simulink model "SimscapePlantModels"  (R2026b)
settings: Solver=VariableStepAuto
undefined symbols (not defined in the file): PlntTrnsfrCaseAxlSpdLock, PlntTrnsfrCaseTrqSplitRatio
libraries: simulink x2, nesl_utility x2
settings Model: ModifiedByFormat=The MathWorks, Inc.  Creator=The MathWorks, Inc.  LastModifiedBy=The MathWorks, Inc.

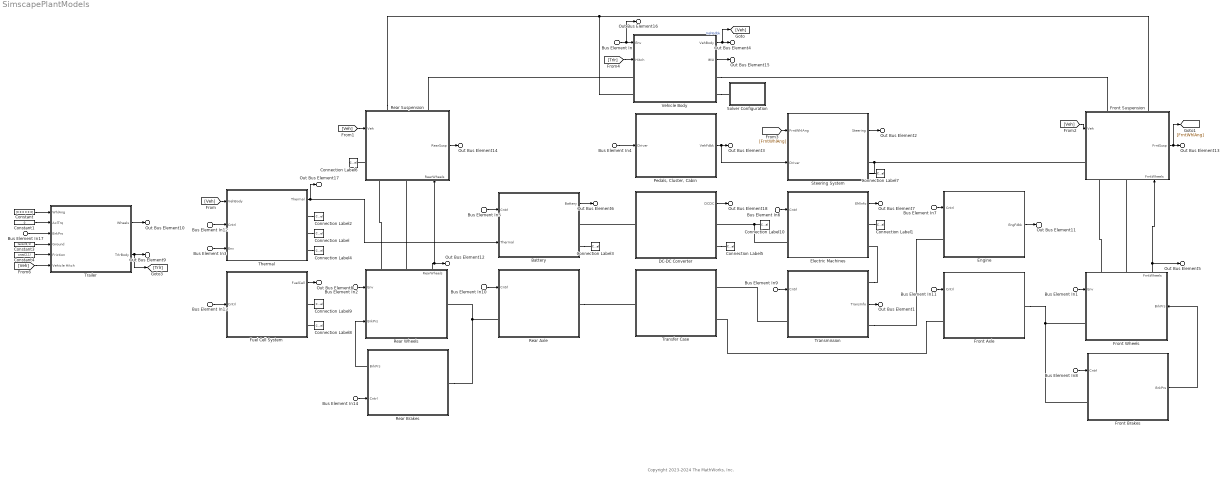
== system SimscapePlantModels ==
  note: Copyright 2023-2024 The MathWorks, Inc.
  Bus Element In{,1..3} (4 alike) : Inport  PortName=Env
  Bus Element In4 : Inport  Port=2  PortName=Driver
  Bus Element In{5..14} (10 alike) : Inport  Port=3  PortName=Cntrl
  Bus Element In17 : Inport  Port=3  PortName=Cntrl  Element=Vcu.VcuTrlrBrkPrsCmd
  Battery : Subsystem  Variant=on  VariantChoicesSpecifier={'BatteryMappedSSC', 'DetailedBatteryModel', 'NoBattery'}  VariantControlMode=label  VariantControl=Battery  LabelModeActiveChoice=NoBattery
      mask Display: image('Battery.png'); % Use "Edit Image" on toolstrip to change.
  Connection Label : ConnectionLabel  Label=ThrmEM
  Connection Label1 : ConnectionLabel  Label=ThrmEM
  Connection Label10 : ConnectionLabel  Label=HVDC
  Connection Label2 : ConnectionLabel  Label=ThrmBatt
  Connection Label3 : ConnectionLabel  Label=ThrmBatt
  Connection Label4 : ConnectionLabel  Label=ThrmPwrE
  Connection Label5 : ConnectionLabel  Label=ThrmPwrE
  Connection Label6 : ConnectionLabel  Label=Steer
  Connection Label7 : ConnectionLabel  Label=Steer
  Connection Label8 : ConnectionLabel  Label=ThrmPwrE
  Connection Label9 : ConnectionLabel  Label=HVDC
  Constant : Constant  Value=[0 0 0 0 0 0]
  Constant1 : Constant  Value=0
  Constant3 : Constant  Value=zeros(2,1)
  Constant4 : Constant  Value=ones(2,1)
  DC-DC Converter : Subsystem  Variant=on  VariantChoicesSpecifier={'DCDCConverterSSC', 'HVDCPassThroughSSC', 'NoDCDCConverter'}  VariantControlMode=label  VariantControl=DC-DC Converter  LabelModeActiveChoice=NoDCDCConverter
      mask Display: image('DCDCConverter.png'); % Use "Edit Image" on toolstrip to change.
  Electric Machines : Subsystem  Variant=on  VariantChoicesSpecifier={'s1EMSSC', 's2EMSSC', 's3EMSSC', 's4EMSSC', 'NoEM'}  VariantControlMode=label  VariantControl=Electric Machines  LabelModeActiveChoice=NoEM
      mask Display: image('Motor.png'); % Use "Edit Image" on toolstrip to change.
  Engine : Subsystem  Variant=on  VariantChoicesSpecifier={'FMUEngineSSC', 'NoEngine', 'SimpleEngineSSC'}  VariantControlMode=label  VariantControl=Engine  LabelModeActiveChoice=SimpleEngineSSC
      settings: PortSchema="{\"entries\":[{\"content\":{\"sides\":[{\"content\":{\"connectorIds\":[\"Out1\"]},\"type\":\"ConnectorPlacement.EquallySpacedRectSide\",\"uuid\":\"a3b8b5c3-27e7-4b20-ab88-ee45fcc797bf\"},{\"content\":{\"connectorIds\":[\"In1\",\"RConn1\"],\"side\":\"RIGHT\"},\"type\":\"ConnectorPlacement.EquallySpacedRectSide\",\"uuid\":\"6bc1f60e-7c62-435c-b993-228d775a2fb7\"},{\"content\":{\"side\":\"TOP\"},\"type\":\"ConnectorPlacement.EquallySpacedRectSide\",\"uuid\":\"10043785-7be0-4314-a245-133c898806ac\"}]},\"type\":\"ConnectorPlacement.EquallySpacedConnector\",\"uuid\":\"16b8f5d8-ca71-4d51-812a-2d43fab8268d\"}],\"packageUris\":[\"http://schema.mathworks.com/mf0/Connector/R2020b\"],\"version\":\"1.0\"}"
      mask Display: image('Engine.png'); % Use "Edit Image" on toolstrip to change.
  Front Axle : Subsystem  Variant=on  VariantChoicesSpecifier={'DualEMDriveFrontSSC', 'LimitedSlipDifferentialSSC', 'NoDifferentialFrontSSC', 'OpenDifferentialSSC'}  VariantControlMode=label  VariantControl=Front Axle  LabelModeActiveChoice=OpenDifferentialSSC
      mask Display: image('Differential.png'); % Use "Edit Image" on toolstrip to change.
  Front Brakes : Subsystem  Variant=on  VariantControlMode=label  LabelModeActiveChoice=BrakingHydraulicsDiscBrakesFrontSSC
      mask Display: image('Caliper.png');
  Front Suspension : Subsystem  Variant=on  VariantChoicesSpecifier={'NoSuspensionFrontSSC', 'MultibodySuspensionFrontSSC'}  VariantControlMode=label  VariantControl=Front Suspension  LabelModeActiveChoice=NoSuspensionFrontSSC
      settings: PortSchema="{\"entries\":[{\"content\":{\"sides\":[{\"content\":{\"connectorIds\":[\"In1\",\"LConn1\"]},\"type\":\"ConnectorPlacement.EquallySpacedRectSide\",\"uuid\":\"36495ae3-e41e-45b1-8235-92554da8a481\"},{\"content\":{\"connectorIds\":[\"Out1\"],\"side\":\"RIGHT\"},\"type\":\"ConnectorPlacement.EquallySpacedRectSide\",\"uuid\":\"e9a47a73-fb93-4125-a24a-a3cc868721b9\"},{\"content\":{\"connectorIds\":[\"LConn2\",\"LConn3\"],\"side\":\"TOP\"},\"type\":\"ConnectorPlacement.EquallySpacedRectSide\",\"uuid\":\"5a383699-364e-4237-a1a1-da409ccbe0dd\"},{\"content\":{\"connectorIds\":[\"RConn1\",\"RConn2\",\"In2\"],\"side\":\"BOTTOM\"},\"type\":\"ConnectorPlacement.EquallySpacedRectSide\",\"uuid\":\"52f047b1-27f7-43e7-8630-25f9b0ada97f\"}]},\"type\":\"ConnectorPlacement.EquallySpacedConnector\",\"uuid\":\"71c041fb-1ceb-419f-94dc-cf2d7d471e97\"}],\"packageUris\":[\"http://schema.mathworks.com/mf0/Connector/R2020b\"],\"version\":\"1.0\"}"
      mask Display: image('SimpleSusp.png'); % Use "Edit Image" on toolstrip to change.
  Front Wheels : Subsystem  Variant=on  VariantChoicesSpecifier={'MFTiresLongitudinalFrontSSC', 'MFTiresMultibodyFrontSSC'}  VariantControlMode=label  VariantControl=Front Wheels  LabelModeActiveChoice=MFTiresLongitudinalFrontSSC
      settings: PortSchema="{\"entries\":[{\"content\":{\"sides\":[{\"content\":{\"connectorIds\":[\"In1\",\"LConn1\"]},\"type\":\"ConnectorPlacement.EquallySpacedRectSide\",\"uuid\":\"18116c41-4c85-4964-ba51-5bd2d68de1c0\"},{\"content\":{\"connectorIds\":[\"In2\"],\"side\":\"RIGHT\"},\"type\":\"ConnectorPlacement.EquallySpacedRectSide\",\"uuid\":\"ed8f79d6-b842-45c2-9629-e45b4856155a\"},{\"content\":{\"connectorIds\":[\"LConn2\",\"LConn3\",\"Out1\"],\"side\":\"TOP\"},\"type\":\"ConnectorPlacement.EquallySpacedRectSide\",\"uuid\":\"6d0f4b93-eb24-4fe5-bb44-e27d25281d66\"}]},\"type\":\"ConnectorPlacement.EquallySpacedConnector\",\"uuid\":\"784a74eb-5e74-45d7-9868-3d9308da2017\"}],\"packageUris\":[\"http://schema.mathworks.com/mf0/Connector/R2020b\"],\"version\":\"1.0\"}"
      mask Display: image('TirewithNoneBrake.png'); % Use "Edit Image" on toolstrip to change.
  Fuel Cell System : Subsystem  Variant=on  VariantControlMode=label  LabelModeActiveChoice=NoFuelCell
  "Pedals, Cluster, Cabin" : Subsystem
  Rear Axle : Subsystem  Variant=on  VariantChoicesSpecifier={'DualEMDriveRear3EMSSC', 'DualEMDriveRear4EMSSC', 'LimitedSlipDifferential2SSC', 'NoDifferentialRearSSC', 'OpenDifferential2SSC'}  VariantControlMode=label  VariantControl=Rear Axle  LabelModeActiveChoice=NoDifferentialRearSSC
      settings: PortSchema="{\"entries\":[{\"content\":{\"sides\":[{\"content\":{\"connectorIds\":[\"LConn1\"]},\"type\":\"ConnectorPlacement.EquallySpacedRectSide\",\"uuid\":\"65d99f67-05a2-47e2-8294-9f529f1023b0\"},{\"content\":{\"connectorIds\":[\"In1\",\"RConn1\"],\"side\":\"RIGHT\"},\"type\":\"ConnectorPlacement.EquallySpacedRectSide\",\"uuid\":\"aa6e28a2-60ee-49c7-b0d1-af08bbc364e9\"},{\"content\":{\"side\":\"TOP\"},\"type\":\"ConnectorPlacement.EquallySpacedRectSide\",\"uuid\":\"5c87d57e-c88d-4b62-ab09-b2529f55e131\"}]},\"type\":\"ConnectorPlacement.EquallySpacedConnector\",\"uuid\":\"05d2764b-b8a6-49cf-a5f1-fcd990b4e9b6\"}],\"packageUris\":[\"http://schema.mathworks.com/mf0/Connector/R2020b\"],\"version\":\"1.0\"}"
      mask Display: image('Differential.png'); % Use "Edit Image" on toolstrip to change.
  Rear Brakes : Subsystem  Variant=on  VariantControlMode=label  LabelModeActiveChoice=BrakingHydraulicsDiscBrakesRearSSC
      settings: PortSchema="{\"entries\":[{\"content\":{\"sides\":[{\"content\":{\"connectorIds\":[\"Out1\",\"In1\"]},\"type\":\"ConnectorPlacement.EquallySpacedRectSide\",\"uuid\":\"1a344f8a-3021-4136-9b8c-8b822c978ed0\"},{\"content\":{\"connectorIds\":[\"RConn1\"],\"side\":\"RIGHT\"},\"type\":\"ConnectorPlacement.EquallySpacedRectSide\",\"uuid\":\"18adbbc3-2fb5-4373-b77a-b21e81530fc9\"},{\"content\":{\"side\":\"TOP\"},\"type\":\"ConnectorPlacement.EquallySpacedRectSide\",\"uuid\":\"fb378fea-1867-4c5a-9e78-cb47ca632c79\"}]},\"type\":\"ConnectorPlacement.EquallySpacedConnector\",\"uuid\":\"a08d4fdb-0a7f-495f-99ba-67ccd9fceaa4\"}],\"packageUris\":[\"http://schema.mathworks.com/mf0/Connector/R2020b\"],\"version\":\"1.0\"}"
      mask Display: image('Caliper.png');
  Rear Suspension : Subsystem  Variant=on  VariantChoicesSpecifier={'NoSuspensionRearSSC', 'MultibodySuspensionRearSSC'}  VariantControlMode=label  VariantControl=Rear Suspension  LabelModeActiveChoice=NoSuspensionRearSSC
      settings: PortSchema="{\"entries\":[{\"content\":{\"sides\":[{\"content\":{\"connectorIds\":[\"In1\",\"LConn1\"]},\"type\":\"ConnectorPlacement.EquallySpacedRectSide\",\"uuid\":\"36495ae3-e41e-45b1-8235-92554da8a481\"},{\"content\":{\"connectorIds\":[\"Out1\"],\"side\":\"RIGHT\"},\"type\":\"ConnectorPlacement.EquallySpacedRectSide\",\"uuid\":\"e9a47a73-fb93-4125-a24a-a3cc868721b9\"},{\"content\":{\"connectorIds\":[\"LConn2\",\"LConn3\"],\"side\":\"TOP\"},\"type\":\"ConnectorPlacement.EquallySpacedRectSide\",\"uuid\":\"5a383699-364e-4237-a1a1-da409ccbe0dd\"},{\"content\":{\"connectorIds\":[\"RConn1\",\"RConn2\",\"In2\"],\"side\":\"BOTTOM\"},\"type\":\"ConnectorPlacement.EquallySpacedRectSide\",\"uuid\":\"f9ad9365-a105-4ce1-87dd-14cbc5e9d7d0\"}]},\"type\":\"ConnectorPlacement.EquallySpacedConnector\",\"uuid\":\"71c041fb-1ceb-419f-94dc-cf2d7d471e97\"}],\"packageUris\":[\"http://schema.mathworks.com/mf0/Connector/R2020b\"],\"version\":\"1.0\"}"
      mask Display: image('SimpleSusp.png'); % Use "Edit Image" on toolstrip to change.
  Rear Wheels : Subsystem  Variant=on  VariantChoicesSpecifier={'MFTiresLongitudinalRearSSC', 'MFTiresMultibodyRearSSC'}  VariantControlMode=label  VariantControl=Rear Wheels  LabelModeActiveChoice=MFTiresLongitudinalRearSSC
      settings: PortSchema="{\"entries\":[{\"content\":{\"sides\":[{\"content\":{\"connectorIds\":[\"LConn1\"]},\"type\":\"ConnectorPlacement.EquallySpacedRectSide\",\"uuid\":\"18116c41-4c85-4964-ba51-5bd2d68de1c0\"},{\"content\":{\"connectorIds\":[\"In1\",\"In2\"],\"side\":\"RIGHT\"},\"type\":\"ConnectorPlacement.EquallySpacedRectSide\",\"uuid\":\"ed8f79d6-b842-45c2-9629-e45b4856155a\"},{\"content\":{\"connectorIds\":[\"Out1\",\"LConn2\",\"LConn3\"],\"side\":\"TOP\"},\"type\":\"ConnectorPlacement.EquallySpacedRectSide\",\"uuid\":\"6d0f4b93-eb24-4fe5-bb44-e27d25281d66\"}]},\"type\":\"ConnectorPlacement.EquallySpacedConnector\",\"uuid\":\"784a74eb-5e74-45d7-9868-3d9308da2017\"}],\"packageUris\":[\"http://schema.mathworks.com/mf0/Connector/R2020b\"],\"version\":\"1.0\"}"
      mask Display: image('TirewithNoneBrake.png'); % Use "Edit Image" on toolstrip to change.
  Solver Configuration : Subsystem  Variant=on  VariantControlMode=label  VariantControl=Choice  LabelModeActiveChoice=Solver Configuration
  Steering System : Subsystem  Variant=on  VariantChoicesSpecifier={'NoSteering', 'SteeringSystemSSC'}  VariantControlMode=label  VariantControl=Steering System  LabelModeActiveChoice=NoSteering
      mask Display: image('SteeringSystemicon.png'); % Use "Edit Image" on toolstrip to change.
  Thermal : Subsystem  Variant=on  VariantChoicesSpecifier={'ElectricalCoolingSystemSSC', 'ElectricalThermalSystemSSC', 'NoThermalEffectSSC'}  VariantControlMode=label  VariantControl=Thermal  LabelModeActiveChoice=NoThermalEffectSSC
      settings: PortSchema="{\"entries\":[{\"content\":{\"sides\":[{\"content\":{\"connectorIds\":[\"Out1\",\"LConn1\",\"LConn2\",\"LConn3\"]},\"type\":\"ConnectorPlacement.EquallySpacedRectSide\",\"uuid\":\"a75df8ce-a1b6-4e8d-bcf9-5e995f514916\"},{\"content\":{\"connectorIds\":[\"In1\",\"In2\",\"In3\"],\"side\":\"RIGHT\"},\"type\":\"ConnectorPlacement.EquallySpacedRectSide\",\"uuid\":\"141082b7-67d4-4180-bfbb-4ef807b696a7\"},{\"content\":{\"side\":\"TOP\"},\"type\":\"ConnectorPlacement.EquallySpacedRectSide\",\"uuid\":\"dccdb1a6-58d5-4cfb-a233-11b972d41f9a\"}]},\"type\":\"ConnectorPlacement.EquallySpacedConnector\",\"uuid\":\"041ca4de-a665-4a80-8ddf-667c21f0ea9b\"}],\"packageUris\":[\"http://schema.mathworks.com/mf0/Connector/R2020b\"],\"version\":\"1.0\"}"
      mask Display: image('ThermalNoFrm.png'); % Use "Edit Image" on toolstrip to change.
  Trailer : Subsystem  Variant=on  VariantChoicesSpecifier={'NoTrailer'}  VariantControlMode=label  VariantControl=No Trailer  LabelModeActiveChoice=NoTrailer
      mask Display: image('6dof1axletrailer.png');
  Transfer Case : Subsystem
      mask Display: image('transfercase.png'); % Use "Edit Image" on toolstrip to change.
  Transmission : Subsystem  Variant=on  VariantChoicesSpecifier={'BEV1EMSSC', 'BEV2EMSSC', 'BEV3EMSSC', 'BEV4EMSSC', 'ConventionalVehicleSSC', 'HEVIPSSSC', 'HEVMMSSC', 'HEVP0SSC', 'HEVP1SSC', 'HEVP2SSC', 'HEVP3SSC', 'HEVP4SSC'}  VariantControlMode=label  VariantControl=Transmission  LabelModeActiveChoice=ConventionalVehicleSSC
      settings: PortSchema="{\"entries\":[{\"content\":{\"sides\":[{\"content\":{\"connectorIds\":[\"LConn1\",\"Out1\",\"LConn2\"]},\"type\":\"ConnectorPlacement.EquallySpacedRectSide\",\"uuid\":\"9098cd8a-1c13-4969-8904-a3c69c3fbea3\"},{\"content\":{\"connectorIds\":[\"In1\",\"RConn1\"],\"side\":\"RIGHT\"},\"type\":\"ConnectorPlacement.EquallySpacedRectSide\",\"uuid\":\"692e5283-fe2f-411a-855c-4b2a88c2de80\"},{\"content\":{\"side\":\"TOP\"},\"type\":\"ConnectorPlacement.EquallySpacedRectSide\",\"uuid\":\"b48dfd83-abc4-4ffd-aa0d-cd09c6e37def\"}]},\"type\":\"ConnectorPlacement.EquallySpacedConnector\",\"uuid\":\"e2c2c99a-9d88-4222-b688-0d6909f509c0\"}],\"packageUris\":[\"http://schema.mathworks.com/mf0/Connector/R2020b\"],\"version\":\"1.0\"}"
      mask Display: image('Transmission.png'); % Use "Edit Image" on toolstrip to change.
  Vehicle Body : Subsystem
      mask Display: image('VehDynLat.png');
  Out Bus Element3 : Outport  PortName=VehFdbk  Element=Driver
  Out Bus Element4 : Outport  PortName=VehFdbk  Element=Body
  Out Bus Element5 : Outport  PortName=VehFdbk  Element=FrntWheels
  Out Bus Element1 : Outport  PortName=VehFdbk  Element=Trans
  Out Bus Element2 : Outport  PortName=VehFdbk  Element=Steering
  Out Bus Element6 : Outport  PortName=VehFdbk  Element=Battery
  Out Bus Element7 : Outport  PortName=VehFdbk  Element=EM
  Out Bus Element8 : Outport  PortName=VehFdbk  Element=FuelCell
  Out Bus Element11 : Outport  PortName=VehFdbk  Element=Engine
  Out Bus Element13 : Outport  PortName=VehFdbk  Element=FrntSuspension
  Out Bus Element9 : Outport  PortName=VehFdbk  Element=TrlrBody
  Out Bus Element10 : Outport  PortName=VehFdbk  Element=TrlrWheels
  Out Bus Element12 : Outport  PortName=VehFdbk  Element=RearWheels
  Out Bus Element14 : Outport  PortName=VehFdbk  Element=RearSuspension
  Out Bus Element15 : Outport  PortName=VehFdbk  Element=IMU
  Out Bus Element16 : Outport  PortName=VehFdbk  Element=Env
  Out Bus Element17 : Outport  PortName=VehFdbk  Element=Thermal
  Out Bus Element18 : Outport  PortName=VehFdbk  Element=DCDC
  wires:
  "Pedals, Cluster, Cabin"/1(VehFdbk) -> Steering System/2(Driver), Out Bus Element3/1
  Front Wheels/1(FrntWheels) -> Front Suspension/2(FrntWheels), Out Bus Element5/1
  Front Suspension/1(FrntSusp) -> [FrntWhlAng], Out Bus Element13/1
  Rear Wheels/1(RearWheels) -> Out Bus Element12/1, Rear Suspension/2(RearWheels)
  Transmission/1(TransInfo) -> Out Bus Element1/1
  Thermal/1(Thermal) -> Out Bus Element17/1, Battery/2(Thermal)
  Bus Element In7/1 -> Engine/1(Cntrl)
  Bus Element In13/1 -> Fuel Cell System/1(Cntrl)
  Engine/1(EngFdbk) -> Out Bus Element11/1
  Vehicle Body/1(VehBody) -> Out Bus Element4/1, [Veh]  "VehFdbk"
  Rear Brakes/1(BrkPrs) -> Rear Wheels/2(BrkPrs)
  Electric Machines/1(EMInfo) -> Out Bus Element7/1
  Steering System/1(Steering) -> Out Bus Element2/1
  Bus Element In2/1 -> Rear Wheels/1(Env)
  Bus Element In/1 -> Vehicle Body/1(Env), Out Bus Element16/1
  Bus Element In4/1 -> "Pedals, Cluster, Cabin"/1(Driver)
  Bus Element In3/1 -> Thermal/3(Env)
  Bus Element In14/1 -> Rear Brakes/1(Cntrl)
  Front Brakes/1(BrkPrs) -> Front Wheels/2(BrkPrs)
  Bus Element In9/1 -> Transmission/1(Cntrl)
  Bus Element In12/1 -> Thermal/2(Cntrl)
  Bus Element In8/1 -> Front Brakes/1(Cntrl)
  Bus Element In5/1 -> Battery/1(Cntrl)
  Rear Suspension/1(RearSusp) -> Out Bus Element14/1
  Fuel Cell System/1(FuelCell) -> Out Bus Element8/1
  Bus Element In6/1 -> Electric Machines/1(Cntrl)
  Bus Element In1/1 -> Front Wheels/1(Env)
  Battery/1(Battery) -> Out Bus Element6/1
  Bus Element In10/1 -> Rear Axle/1(Cntrl)
  Bus Element In11/1 -> Front Axle/1(Cntrl)
  Vehicle Body/2(IMU) -> Out Bus Element15/1
  [Veh] -> Rear Suspension/1(Veh)
  [Veh] -> Front Suspension/1(Veh)
  [FrntWhlAng] -> Steering System/1(FrntWhlAng)
  [Trlr] -> Vehicle Body/2(Hitch)
  DC-DC Converter/1(DCDC) -> Out Bus Element18/1
  Trailer/2(TrlrBody) -> [Trlr], Out Bus Element9/1
  [Veh] -> Trailer/6(Vehicle Hitch)
  Bus Element In17/1 -> Trailer/3(BrkPrs)
  Constant/1 -> Trailer/1(WhlAng)
  Constant3/1 -> Trailer/4(Ground)
  Constant4/1 -> Trailer/5(Friction)
  Constant1/1 -> Trailer/2(AxlTrq)
  Trailer/1(Wheels) -> Out Bus Element10/1
  [Veh] -> Thermal/1(VehBody)
  connections:
  Rear Suspension/LConn2 -- Front Suspension/LConn3 -- Vehicle Body/LConn2
  Rear Brakes/RConn1 -- Rear Wheels/LConn1 -- Rear Axle/RConn1
  Front Brakes/LConn1 -- Front Wheels/LConn1 -- Front Axle/RConn1
  DC-DC Converter/RConn1 -- Electric Machines/LConn1 -- Connection Label10/LConn1
  Connection Label7/LConn1 -- Steering System/RConn1 -- Front Suspension/LConn1
  Fuel Cell System/RConn1 -- Connection Label9/LConn1
  Connection Label8/LConn1 -- Fuel Cell System/RConn2
  Thermal/LConn1 -- Connection Label2/LConn1
  Transmission/LConn1 -- Electric Machines/RConn2
  Front Axle/LConn1 -- Transfer Case/RConn2
  Rear Suspension/LConn3 -- Vehicle Body/LConn1
  Thermal/LConn2 -- Connection Label/LConn1
  Thermal/LConn3 -- Connection Label4/LConn1
  Electric Machines/RConn1 -- Connection Label1/LConn1
  Rear Wheels/LConn3 -- Rear Suspension/RConn1
  Rear Suspension/LConn1 -- Connection Label6/LConn1
  DC-DC Converter/LConn1 -- Battery/RConn1
  Transmission/LConn2 -- Engine/RConn1
  DC-DC Converter/RConn2 -- Connection Label5/LConn1
  Battery/RConn2 -- Connection Label3/LConn1
  Front Wheels/LConn2 -- Front Suspension/RConn1
  Rear Axle/LConn1 -- Transfer Case/LConn1
  Vehicle Body/RConn2 -- Solver Configuration/RConn1
  Vehicle Body/RConn1 -- Front Suspension/LConn2
  Transmission/RConn1 -- Transfer Case/RConn1
  Front Wheels/LConn3 -- Front Suspension/RConn2
  Rear Wheels/LConn2 -- Rear Suspension/RConn2

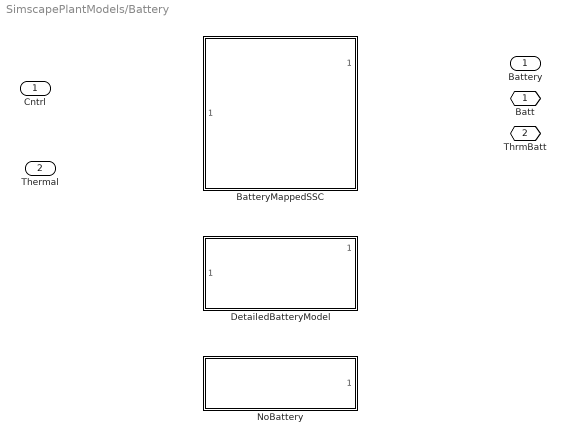
== system SimscapePlantModels/Battery ==
  Cntrl : Inport
  Thermal : Inport  Port=2
  BatteryMappedSSC : Subsystem  VariantControl=BatteryMappedSSC  ReferencedSubsystem=BatteryMappedSSC
  DetailedBatteryModel : Subsystem  VariantControl=DetailedBatteryModel  ReferencedSubsystem=DetailedBatteryModel
  NoBattery : Subsystem  VariantControl=NoBattery  ReferencedSubsystem=NoBattery
  Batt : PMIOPort  Side=Right
  ThrmBatt : PMIOPort  Port=2  Side=Right
  Battery : Outport

== system SimscapePlantModels/DC-DC Converter ==
  DCDCConverterSSC : Subsystem  VariantControl=DCDCConverterSSC  ReferencedSubsystem=DCDCConverterSSC
  HVDCPassThroughSSC : Subsystem  VariantControl=HVDCPassThroughSSC  ReferencedSubsystem=HVDCPassThroughSSC
  NoDCDCConverter : Subsystem  VariantControl=NoDCDCConverter  ReferencedSubsystem=NoDCDCConverter
  Batt : PMIOPort  Side=Left
  HVDC : PMIOPort  Port=2  Side=Right
  ThrmPwrE : PMIOPort  Port=3  Side=Right
  DCDC : Outport

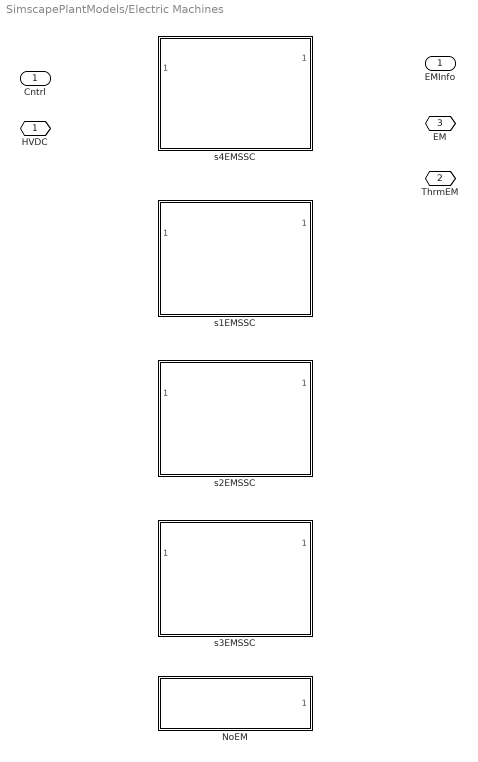
== system SimscapePlantModels/Electric Machines ==
  Cntrl : Inport
  NoEM : Subsystem  VariantControl=NoEM  ReferencedSubsystem=NoEM
  s1EMSSC : Subsystem  VariantControl=s1EMSSC  ReferencedSubsystem=s1EMSSC
  s2EMSSC : Subsystem  VariantControl=s2EMSSC  ReferencedSubsystem=s2EMSSC
  s3EMSSC : Subsystem  VariantControl=s3EMSSC  ReferencedSubsystem=s3EMSSC
  s4EMSSC : Subsystem  VariantControl=s4EMSSC  ReferencedSubsystem=s4EMSSC
  HVDC : PMIOPort  Side=Left
  ThrmEM : PMIOPort  Port=2  Side=Right
  EM : PMIOPort  Port=3  Side=Right
  EMInfo : Outport

== system SimscapePlantModels/Engine ==
  Cntrl : Inport
  FMUEngineSSC : Subsystem  VariantControl=FMUEngineSSC  ReferencedSubsystem=FMUEngineSSC
  NoEngine : Subsystem  VariantControl=NoEngine  ReferencedSubsystem=NoEngine
  SimpleEngineSSC : Subsystem  VariantControl=SimpleEngineSSC  ReferencedSubsystem=SimpleEngineSSC
  EngTrq : PMIOPort  Side=Right
  EngFdbk : Outport

== system SimscapePlantModels/Front Axle ==
  Cntrl : Inport
  DualEMDriveFrontSSC : Subsystem  VariantControl=DualEMDriveFrontSSC  ReferencedSubsystem=DualEMDriveFrontSSC
  LimitedSlipDifferentialSSC : Subsystem  VariantControl=LimitedSlipDifferentialSSC  ReferencedSubsystem=LimitedSlipDifferentialSSC
  NoDifferentialFrontSSC : Subsystem  VariantControl=NoDifferentialFrontSSC  ReferencedSubsystem=NoDifferentialFrontSSC
  OpenDifferentialSSC : Subsystem  VariantControl=OpenDifferentialSSC  ReferencedSubsystem=OpenDifferentialSSC
  DriveshftTrq : PMIOPort  Side=Left
  AxlTrq : PMIOPort  Port=2  Side=Right

== system SimscapePlantModels/Front Brakes ==
  Cntrl : Inport
  BrakingHydraulicsDiscBrakesFrontSSC : Subsystem  VariantControl=BrakingHydraulicsDiscBrakesFrontSSC  ReferencedSubsystem=BrakingHydraulicsDiscBrakesFrontSSC
  Axl : PMIOPort  Side=Left
  BrkPrs : Outport

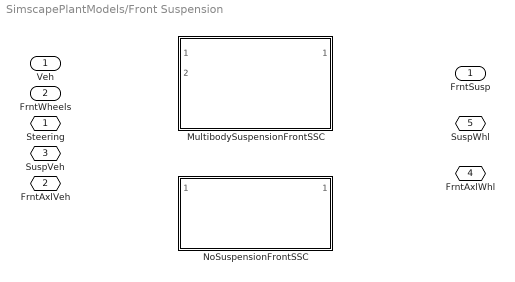
== system SimscapePlantModels/Front Suspension ==
  Veh : Inport
  FrntWheels : Inport  Port=2
  MultibodySuspensionFrontSSC : Subsystem  VariantControl=MultibodySuspensionFrontSSC  ReferencedSubsystem=MultibodySuspensionFrontSSC
  NoSuspensionFrontSSC : Subsystem  VariantControl=NoSuspensionFrontSSC  ReferencedSubsystem=NoSuspensionFrontSSC
  Steering : PMIOPort  Side=Left
  FrntAxlVeh : PMIOPort  Port=2  Side=Left
  SuspVeh : PMIOPort  Port=3  Side=Left
  FrntAxlWhl : PMIOPort  Port=4  Side=Right
  SuspWhl : PMIOPort  Port=5  Side=Right
  FrntSusp : Outport

== system SimscapePlantModels/Front Wheels ==
  Env : Inport
  BrkPrs : Inport  Port=2
  MFTiresLongitudinalFrontSSC : Subsystem  VariantControl=MFTiresLongitudinalFrontSSC  ReferencedSubsystem=MFTiresLongitudinalFrontSSC
  MFTiresMultibodyFrontSSC : Subsystem  VariantControl=MFTiresMultibodyFrontSSC  ReferencedSubsystem=MFTiresMultibodyFrontSSC
  Axl : PMIOPort  Side=Left
  FrntAxlWhl : PMIOPort  Port=2  Side=Left
  SuspWhl : PMIOPort  Port=3  Side=Left
  FrntWheels : Outport

== system SimscapePlantModels/Fuel Cell System ==
  Cntrl : Inport
  FuelCellSSC : Subsystem  VariantControl=FuelCellSSC  ReferencedSubsystem=FuelCellSSC
  NoFuelCell : Subsystem  VariantControl=NoFuelCell  ReferencedSubsystem=NoFuelCell
  HVDC : PMIOPort  Side=Right
  H : PMIOPort  Port=2  Side=Right
  FuelCell : Outport

== system SimscapePlantModels/Pedals, Cluster, Cabin ==
  Driver : Inport
  Pedal Cluster Input : Subsystem
  "Pedal, Cluster, Cabin" : Subsystem
  VehFdbk : Outport
  wires:
  Pedal Cluster Input/1(SteerCmd) -> "Pedal, Cluster, Cabin"/1(SteerCmd)
  Pedal Cluster Input/2(AccelCmd) -> "Pedal, Cluster, Cabin"/2(AccCmd)
  Pedal Cluster Input/3(DecelCmd) -> "Pedal, Cluster, Cabin"/3(DecelCmd)
  Pedal Cluster Input/4(DrvrGearCmd) -> "Pedal, Cluster, Cabin"/4(GearCmd)
  Pedal Cluster Input/5(IgnCmd) -> "Pedal, Cluster, Cabin"/5(IgCmd)
  Pedal Cluster Input/6(HighBeamCmd) -> "Pedal, Cluster, Cabin"/6(HighBeamCmd)
  Pedal Cluster Input/7(LowBeamCmd) -> "Pedal, Cluster, Cabin"/7(LowBeamCmd)
  Pedal Cluster Input/8(LeftSignalCmd) -> "Pedal, Cluster, Cabin"/8(LeftSignalCmd)
  Pedal Cluster Input/9(RightSignalCmd) -> "Pedal, Cluster, Cabin"/9(RightSignalCmd)
  Pedal Cluster Input/10(HazzardCmd) -> "Pedal, Cluster, Cabin"/10(HazzardCmd)
  Driver/1 -> Pedal Cluster Input/1(Driver)
  "Pedal, Cluster, Cabin"/1(Driver) -> VehFdbk/1

== system SimscapePlantModels/Rear Axle ==
  Cntrl : Inport
  DualEMDriveRear3EMSSC : Subsystem  VariantControl=DualEMDriveRear3EMSSC  ReferencedSubsystem=DualEMDriveRear3EMSSC
  DualEMDriveRear4EMSSC : Subsystem  VariantControl=DualEMDriveRear4EMSSC  ReferencedSubsystem=DualEMDriveRear4EMSSC
  LimitedSlipDifferential2SSC : Subsystem  VariantControl=LimitedSlipDifferential2SSC  ReferencedSubsystem=LimitedSlipDifferential2SSC
  NoDifferentialRearSSC : Subsystem  VariantControl=NoDifferentialRearSSC  ReferencedSubsystem=NoDifferentialRearSSC
  OpenDifferential2SSC : Subsystem  VariantControl=OpenDifferential2SSC  ReferencedSubsystem=OpenDifferential2SSC
  DriveshftTrq : PMIOPort  Side=Left
  AxlTrq : PMIOPort  Port=2  Side=Right

== system SimscapePlantModels/Rear Brakes ==
  Cntrl : Inport
  BrakingHydraulicsDiscBrakesRearSSC : Subsystem  VariantControl=BrakingHydraulicsDiscBrakesRearSSC  ReferencedSubsystem=BrakingHydraulicsDiscBrakesRearSSC
  Axl : PMIOPort  Side=Right
  BrkPrs : Outport

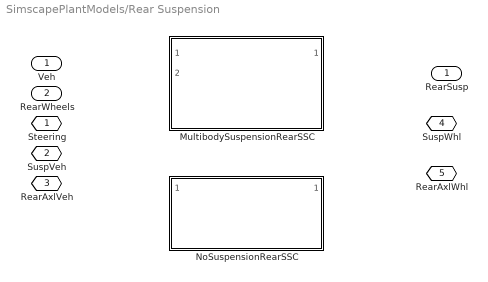
== system SimscapePlantModels/Rear Suspension ==
  Veh : Inport
  RearWheels : Inport  Port=2
  MultibodySuspensionRearSSC : Subsystem  VariantControl=MultibodySuspensionRearSSC  ReferencedSubsystem=MultibodySuspensionRearSSC
  NoSuspensionRearSSC : Subsystem  VariantControl=NoSuspensionRearSSC  ReferencedSubsystem=NoSuspensionRearSSC
  Steering : PMIOPort  Side=Left
  SuspVeh : PMIOPort  Port=2  Side=Left
  RearAxlVeh : PMIOPort  Port=3  Side=Left
  SuspWhl : PMIOPort  Port=4  Side=Right
  RearAxlWhl : PMIOPort  Port=5  Side=Right
  RearSusp : Outport

== system SimscapePlantModels/Rear Wheels ==
  Env : Inport
  BrkPrs : Inport  Port=2
  MFTiresLongitudinalRearSSC : Subsystem  VariantControl=MFTiresLongitudinalRearSSC  ReferencedSubsystem=MFTiresLongitudinalRearSSC
  MFTiresMultibodyRearSSC : Subsystem  VariantControl=MFTiresMultibodyRearSSC  ReferencedSubsystem=MFTiresMultibodyRearSSC
  Axl : PMIOPort  Side=Left
  RearAxlWhl : PMIOPort  Port=2  Side=Left
  SuspWhl : PMIOPort  Port=3  Side=Left
  RearWheels : Outport

== system SimscapePlantModels/Solver Configuration ==
  Local Solver : nesl_utility/Solver Configuration  VariantControl=Local Solver  PhysicalDomain=network_engine_domain  SubClassName=solver  LeftPortType=input  RightPortType=generic  Tones=[]  Harmonics=[]  SimulateNoise=off  Profile=off  UseLocalSampling=off  EnableSwitchedLinearOptims=on  FrequencyDomain=off  UseCCode=off  RelTol=0.001  AbsTol=0.001  MinStep=1e-09  ToWorkspace=off  RevertToSquareIcSolve=off  NumHomotopyIterations=100  PhasorMode=off  PhasorModeNumHarmonics=1  ConsistencySolver=NEWTON_XTOL_AFTER_FTOL  CanonicalOrdering=UNORDERED  OptimizeIntermediates=UNOPTIMIZED  MulticoreSolverChoice=BACKWARD_EULER  IndexReductionMethod=DerivativeReplacement  DoDC=off  ResidualTolerance=1e-09  ConsistencyTolSource=LOCAL  ConsistencyAbsTol=0.001  ConsistencyRelTol=0.001  ConsistencyTolFactor=0.001  UseLocalSolver=on  LocalSolverChoice=NE_BACKWARD_EULER_ADVANCER  ResolveIndetEquations=on  FunctionEvalNumThread=1  LocalSolverSampleTime=0.1  DoFixedCost=off  MaxNonlinIter=3  MaxModeIter=2  ComputeImpulses=off  ImpulseIterations=2  LinearAlgebra=auto  LinearAlgebraNumThread=0  EquationFormulation=NE_TIME_EF  DelaysMemoryBudget=1024  AutomaticFiltering=on  FilteringTimeConstant=0.001  PartitionStorageMethod=AS_NEEDED  PartitionMemoryBudget=1024  PartitionMethod=BALANCED  MultibodyUseLocalSolver=off  MultibodyLocalSolverChoice=ODE1  MultibodyLocalSolverSampleTime=0.001
  Solver Configuration : nesl_utility/Solver Configuration  VariantControl=Solver Configuration  PhysicalDomain=network_engine_domain  SubClassName=solver  LeftPortType=input  RightPortType=generic  Tones=[]  Harmonics=[]  SimulateNoise=off  Profile=off  UseLocalSampling=off  EnableSwitchedLinearOptims=on  FrequencyDomain=off  UseCCode=off  RelTol=0.001  AbsTol=0.001  MinStep=1e-09  ToWorkspace=off  RevertToSquareIcSolve=off  NumHomotopyIterations=100  PhasorMode=off  PhasorModeNumHarmonics=1  ConsistencySolver=NEWTON_XTOL_AFTER_FTOL  CanonicalOrdering=UNORDERED  OptimizeIntermediates=UNOPTIMIZED  MulticoreSolverChoice=BACKWARD_EULER  IndexReductionMethod=DerivativeReplacement  DoDC=off  ResidualTolerance=1e-09  ConsistencyTolSource=LOCAL  ConsistencyAbsTol=0.001  ConsistencyRelTol=0.001  ConsistencyTolFactor=0.001  UseLocalSolver=off  LocalSolverChoice=NE_BACKWARD_EULER_ADVANCER  ResolveIndetEquations=on  FunctionEvalNumThread=1  LocalSolverSampleTime=0.001  DoFixedCost=off  MaxNonlinIter=3  MaxModeIter=2  ComputeImpulses=off  ImpulseIterations=2  LinearAlgebra=auto  LinearAlgebraNumThread=0  EquationFormulation=NE_TIME_EF  DelaysMemoryBudget=1024  AutomaticFiltering=on  FilteringTimeConstant=0.001  PartitionStorageMethod=AS_NEEDED  PartitionMemoryBudget=1024  PartitionMethod=BALANCED  MultibodyUseLocalSolver=off  MultibodyLocalSolverChoice=ODE1  MultibodyLocalSolverSampleTime=0.001
  port : PMIOPort  Side=Right

== system SimscapePlantModels/Steering System ==
  FrntWhlAng : Inport
  Driver : Inport  Port=2
  NoSteering : Subsystem  VariantControl=NoSteering  ReferencedSubsystem=NoSteering
  SteeringSystemSSC : Subsystem  VariantControl=SteeringSystemSSC  ReferencedSubsystem=SteeringSystemSSC
  SteerSusp : PMIOPort  Side=Right
  Steering : Outport

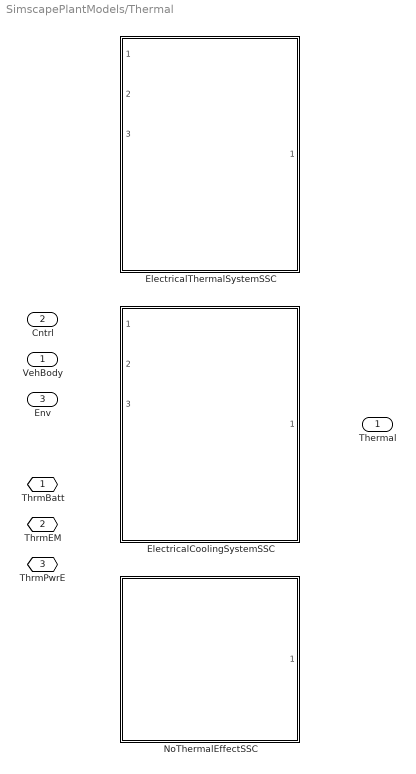
== system SimscapePlantModels/Thermal ==
  VehBody : Inport
  Cntrl : Inport  Port=2
  Env : Inport  Port=3
  ElectricalCoolingSystemSSC : Subsystem  VariantControl=ElectricalCoolingSystemSSC  ReferencedSubsystem=ElectricalCoolingSystemSSC
  ElectricalThermalSystemSSC : Subsystem  VariantControl=ElectricalThermalSystemSSC  ReferencedSubsystem=ElectricalThermalSystemSSC
  NoThermalEffectSSC : Subsystem  VariantControl=NoThermalEffectSSC  ReferencedSubsystem=NoThermalEffectSSC
  ThrmBatt : PMIOPort  Side=Left
  ThrmEM : PMIOPort  Port=2  Side=Left
  ThrmPwrE : PMIOPort  Port=3  Side=Left
  Thermal : Outport

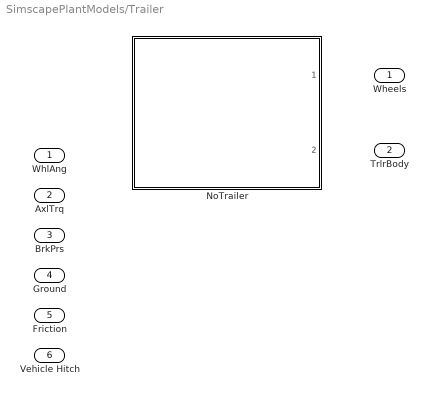
== system SimscapePlantModels/Trailer ==
  WhlAng : Inport
  AxlTrq : Inport  Port=2
  BrkPrs : Inport  Port=3
  Ground : Inport  Port=4
  Friction : Inport  Port=5
  Vehicle Hitch : Inport  Port=6
  NoTrailer : Subsystem  VariantControl=NoTrailer  ReferencedSubsystem=NoTrailer
  Wheels : Outport
  TrlrBody : Outport  Port=2

== system SimscapePlantModels/Transfer Case ==
  Axle Interconnect : Subsystem  Variant=on  VariantChoicesSpecifier={'NoInterconnectSSC', 'TransferCaseSSC'}  VariantControlMode=label  VariantControl=Choice  LabelModeActiveChoice=NoInterconnectSSC
  Constant : Constant  Value=PlntTrnsfrCaseTrqSplitRatio  SampleTime=-1
  Constant1 : Constant  Value=PlntTrnsfrCaseAxlSpdLock  SampleTime=-1
  DriveshftTrq Routing : Subsystem  Variant=on  VariantChoicesSpecifier={'FourActuatorAWDSSC', 'OneActuatorAWDSSC', 'OneActuatorFWDSSC', 'OneActuatorRWDSSC', 'ThreeActuatorAWD2EMFrontSSC', 'ThreeActuatorAWD2EMRearSSC', 'TwoActuatorAWDSSC'}  VariantControlMode=label  VariantControl=Choice  LabelModeActiveChoice=OneActuatorFWDSSC
  Terminator : Terminator
  DriveshftTrq : PMIOPort  Side=Right
  FrntDiffrntlTrq : PMIOPort  Port=2  Side=Right
  RearDiffrntlTrq : PMIOPort  Port=3  Side=Left
  wires:
  DriveshftTrq Routing/1(DriveshftSpd) -> Terminator/1
  Constant1/1 -> Axle Interconnect/2(Lockup)
  Constant/1 -> Axle Interconnect/1(SplitRatio)
  connections:
  RearDiffrntlTrq/RConn1 -- DriveshftTrq Routing/RConn5
  Axle Interconnect/LConn2 -- DriveshftTrq Routing/RConn3
  Axle Interconnect/LConn3 -- DriveshftTrq Routing/RConn4
  Axle Interconnect/LConn1 -- DriveshftTrq Routing/RConn2
  DriveshftTrq/RConn1 -- DriveshftTrq Routing/LConn1
  DriveshftTrq Routing/RConn1 -- FrntDiffrntlTrq/RConn1

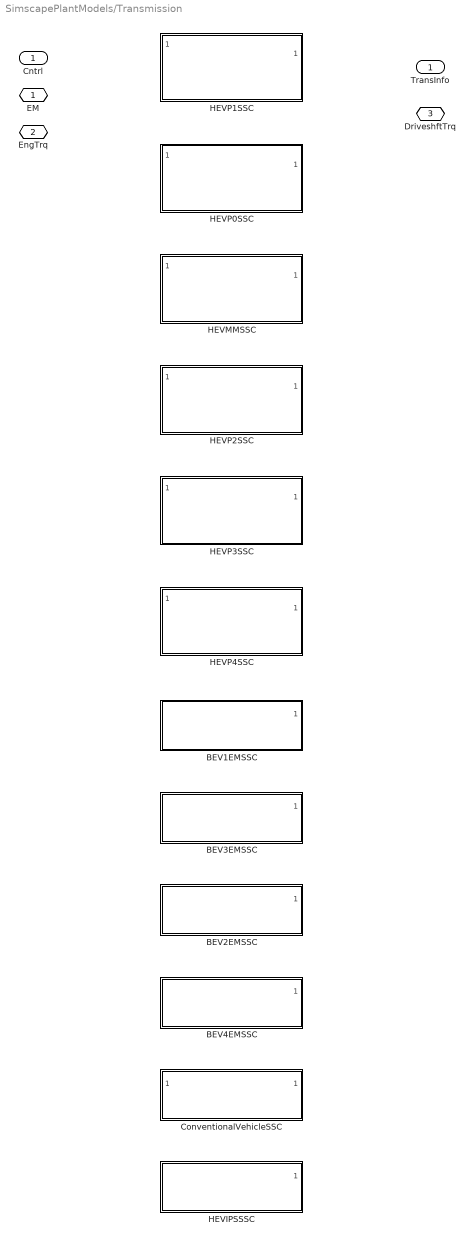
== system SimscapePlantModels/Transmission ==
  Cntrl : Inport
  BEV1EMSSC : Subsystem  VariantControl=BEV1EMSSC  ReferencedSubsystem=BEV1EMSSC
  BEV2EMSSC : Subsystem  VariantControl=BEV2EMSSC  ReferencedSubsystem=BEV2EMSSC
  BEV3EMSSC : Subsystem  VariantControl=BEV3EMSSC  ReferencedSubsystem=BEV3EMSSC
  BEV4EMSSC : Subsystem  VariantControl=BEV4EMSSC  ReferencedSubsystem=BEV4EMSSC
  ConventionalVehicleSSC : Subsystem  VariantControl=ConventionalVehicleSSC  ReferencedSubsystem=ConventionalVehicleSSC
  HEVIPSSSC : Subsystem  VariantControl=HEVIPSSSC  ReferencedSubsystem=HEVIPSSSC
  HEVMMSSC : Subsystem  VariantControl=HEVMMSSC  ReferencedSubsystem=HEVMMSSC
  HEVP0SSC : Subsystem  VariantControl=HEVP0SSC  ReferencedSubsystem=HEVP0SSC
  HEVP1SSC : Subsystem  VariantControl=HEVP1SSC  ReferencedSubsystem=HEVP1SSC
  HEVP2SSC : Subsystem  VariantControl=HEVP2SSC  ReferencedSubsystem=HEVP2SSC
  HEVP3SSC : Subsystem  VariantControl=HEVP3SSC  ReferencedSubsystem=HEVP3SSC
  HEVP4SSC : Subsystem  VariantControl=HEVP4SSC  ReferencedSubsystem=HEVP4SSC
  EM : PMIOPort  Side=Left
  EngTrq : PMIOPort  Port=2  Side=Left
  DriveshftTrq : PMIOPort  Port=3  Side=Right
  TransInfo : Outport

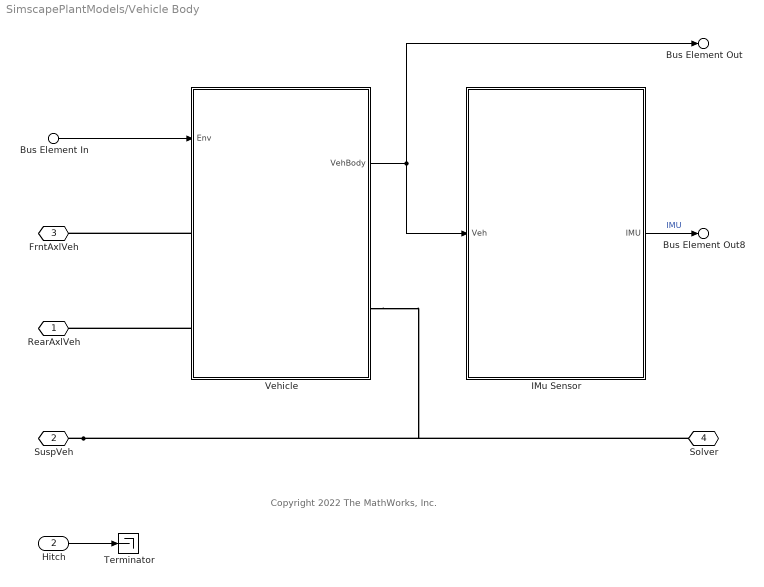
== system SimscapePlantModels/Vehicle Body ==
  note: Copyright 2022 The MathWorks, Inc.
  Bus Element In : Inport  PortName=Env
  Hitch : Inport  Port=2
  IMu Sensor : Subsystem  Variant=on  VariantChoicesSpecifier={'IMUSensor', 'NoIMUSensor'}  VariantControlMode=label  VariantControl=Choice  LabelModeActiveChoice=NoIMUSensor
  Terminator : Terminator
  Vehicle : Subsystem  Variant=on  VariantChoicesSpecifier={'VehicleBody1DOFLongitudinalSSC', 'VehicleBody2DOFLongitudinalSSC', 'VehicleBody6DOFSSC'}  VariantControlMode=label  VariantControl=Vehicle  LabelModeActiveChoice=VehicleBody2DOFLongitudinalSSC
  RearAxlVeh : PMIOPort  Side=Left
  SuspVeh : PMIOPort  Port=2  Side=Left
  FrntAxlVeh : PMIOPort  Port=3  Side=Right
  Solver : PMIOPort  Port=4  Side=Right
  Bus Element Out : Outport  PortName=VehBody
  Bus Element Out8 : Outport  Port=2  PortName=IMU
  wires:
  Hitch/1 -> Terminator/1
  Vehicle/1(VehBody) -> IMu Sensor/1(Veh), Bus Element Out/1
  Bus Element In/1 -> Vehicle/1(Env)
  IMu Sensor/1(IMU) -> Bus Element Out8/1  "IMU"
  connections:
  SuspVeh/RConn1 -- Solver/RConn1 -- Vehicle/RConn1
  Vehicle/LConn2 -- RearAxlVeh/RConn1
  Vehicle/LConn1 -- FrntAxlVeh/RConn1

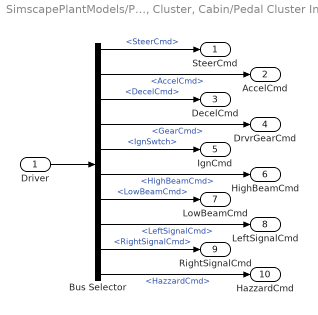
== system SimscapePlantModels/Pedals, Cluster, Cabin/Pedal Cluster Input ==
  Driver : Inport
  Bus Selector : BusSelector  OutputSignals=SteerCmd,AccelCmd,DecelCmd,GearCmd,IgnSwtch,LightsCmd.HighBeamCmd,LightsCmd.LowBeamCmd,LightsCmd.LeftSignalCmd,LightsCmd.RightSignalCmd,LightsCmd.HazzardCmd
  SteerCmd : Outport  VectorParamsAs1DForOutWhenUnconnected=off
  AccelCmd : Outport  Port=2  VectorParamsAs1DForOutWhenUnconnected=off
  DecelCmd : Outport  Port=3  VectorParamsAs1DForOutWhenUnconnected=off
  DrvrGearCmd : Outport  Port=4  VectorParamsAs1DForOutWhenUnconnected=off
  IgnCmd : Outport  Port=5  VectorParamsAs1DForOutWhenUnconnected=off
  HighBeamCmd : Outport  Port=6  VectorParamsAs1DForOutWhenUnconnected=off
  LowBeamCmd : Outport  Port=7  VectorParamsAs1DForOutWhenUnconnected=off
  LeftSignalCmd : Outport  Port=8  VectorParamsAs1DForOutWhenUnconnected=off
  RightSignalCmd : Outport  Port=9  VectorParamsAs1DForOutWhenUnconnected=off
  HazzardCmd : Outport  Port=10  VectorParamsAs1DForOutWhenUnconnected=off
  wires:
  Bus Selector/10 -> HazzardCmd/1  "<HazzardCmd>"
  Bus Selector/9 -> RightSignalCmd/1  "<RightSignalCmd>"
  Bus Selector/8 -> LeftSignalCmd/1  "<LeftSignalCmd>"
  Bus Selector/7 -> LowBeamCmd/1  "<LowBeamCmd>"
  Bus Selector/6 -> HighBeamCmd/1  "<HighBeamCmd>"
  Bus Selector/5 -> IgnCmd/1  "<IgnSwtch>"
  Bus Selector/1 -> SteerCmd/1  "<SteerCmd>"
  Bus Selector/4 -> DrvrGearCmd/1  "<GearCmd>"
  Bus Selector/3 -> DecelCmd/1  "<DecelCmd>"
  Driver/1 -> Bus Selector/1
  Bus Selector/2 -> AccelCmd/1  "<AccelCmd>"

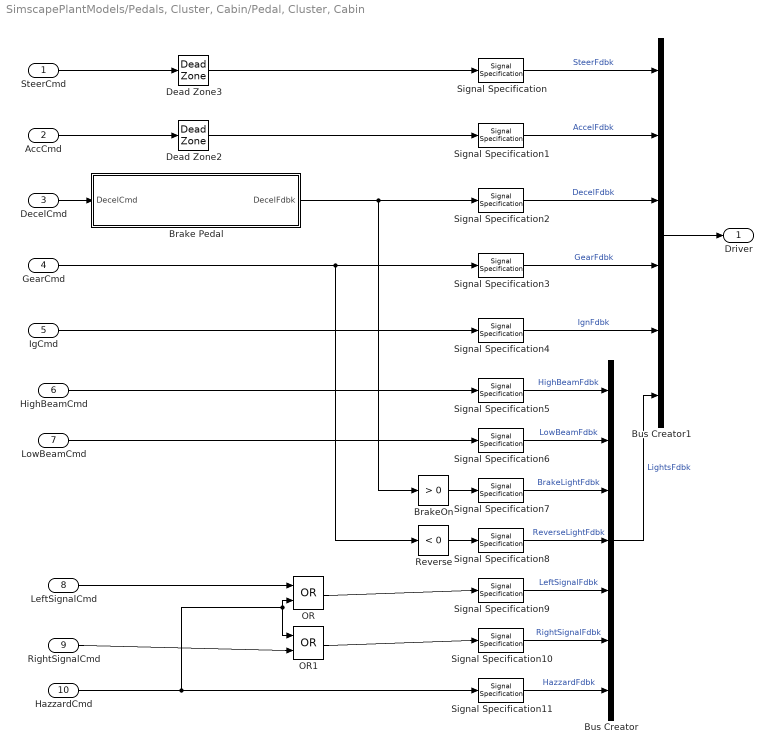
== system SimscapePlantModels/Pedals, Cluster, Cabin/Pedal, Cluster, Cabin ==
  SteerCmd : Inport
  AccCmd : Inport  Port=2
  DecelCmd : Inport  Port=3
  GearCmd : Inport  Port=4
  IgCmd : Inport  Port=5
  HighBeamCmd : Inport  Port=6
  LowBeamCmd : Inport  Port=7
  LeftSignalCmd : Inport  Port=8
  RightSignalCmd : Inport  Port=9
  HazzardCmd : Inport  Port=10
  Brake Pedal : Subsystem
  BrakeOn : simulink/Logic and Bit Operations/Compare To Constant  relop=>  const=0  OutDataTypeStr=boolean  ZeroCross=off
  Bus Creator : BusCreator  Inputs=7
  Bus Creator1 : BusCreator  Inputs=6
  Dead Zone2 : DeadZone  LowerValue=0  UpperValue=.01  ZeroCross=off
  Dead Zone3 : DeadZone  LowerValue=-.01  UpperValue=.01  ZeroCross=off
  OR : Logic  Operator=OR  IconShape=distinctive  AllPortsSameDT=off  OutDataTypeStr=boolean
  OR1 : Logic  Operator=OR  IconShape=distinctive  AllPortsSameDT=off  OutDataTypeStr=boolean
  Reverse : simulink/Logic and Bit Operations/Compare To Constant  relop=<  const=0  OutDataTypeStr=boolean  ZeroCross=off
  Signal Specification : SignalSpecification  Unit=rad
  Signal Specification{1..11} (11 alike) : SignalSpecification  Unit=1
  Driver : Outport
  wires:
  Signal Specification9/1 -> Bus Creator/5  "LeftSignalFdbk"
  Signal Specification11/1 -> Bus Creator/7  "HazzardFdbk"
  Signal Specification10/1 -> Bus Creator/6  "RightSignalFdbk"
  Signal Specification8/1 -> Bus Creator/4  "ReverseLightFdbk"
  Signal Specification7/1 -> Bus Creator/3  "BrakeLightFdbk"
  Signal Specification6/1 -> Bus Creator/2  "LowBeamFdbk"
  Signal Specification5/1 -> Bus Creator/1  "HighBeamFdbk"
  Bus Creator/1 -> Bus Creator1/6  "LightsFdbk"
  RightSignalCmd/1 -> OR1/2
  LowBeamCmd/1 -> Signal Specification6/1
  HazzardCmd/1 -> OR1/1, OR/2, Signal Specification11/1
  LeftSignalCmd/1 -> OR/1
  Reverse/1 -> Signal Specification8/1
  OR/1 -> Signal Specification9/1
  OR1/1 -> Signal Specification10/1
  BrakeOn/1 -> Signal Specification7/1
  HighBeamCmd/1 -> Signal Specification5/1
  Dead Zone3/1 -> Signal Specification/1
  Signal Specification1/1 -> Bus Creator1/2  "AccelFdbk"
  Signal Specification4/1 -> Bus Creator1/5  "IgnFdbk"
  Brake Pedal/1(DecelFdbk) -> Signal Specification2/1, BrakeOn/1
  Signal Specification/1 -> Bus Creator1/1  "SteerFdbk"
  Signal Specification2/1 -> Bus Creator1/3  "DecelFdbk"
  GearCmd/1 -> Signal Specification3/1, Reverse/1
  Bus Creator1/1 -> Driver/1
  IgCmd/1 -> Signal Specification4/1
  Signal Specification3/1 -> Bus Creator1/4  "GearFdbk"
  Dead Zone2/1 -> Signal Specification1/1
  SteerCmd/1 -> Dead Zone3/1
  AccCmd/1 -> Dead Zone2/1
  DecelCmd/1 -> Brake Pedal/1(DecelCmd)

== system SimscapePlantModels/Transfer Case/Axle Interconnect ==
  SplitRatio : Inport
  Lockup : Inport  Port=2
  NoInterconnectSSC : Subsystem  VariantControl=NoInterconnectSSC  ReferencedSubsystem=NoInterconnectSSC
  TransferCaseSSC : Subsystem  VariantControl=TransferCaseSSC  ReferencedSubsystem=TransferCaseSSC
  FrntDiffrntlTrq : PMIOPort  Side=Left
  DriveshftTrq : PMIOPort  Port=2  Side=Left
  RearDiffrntlTrq : PMIOPort  Port=3  Side=Left

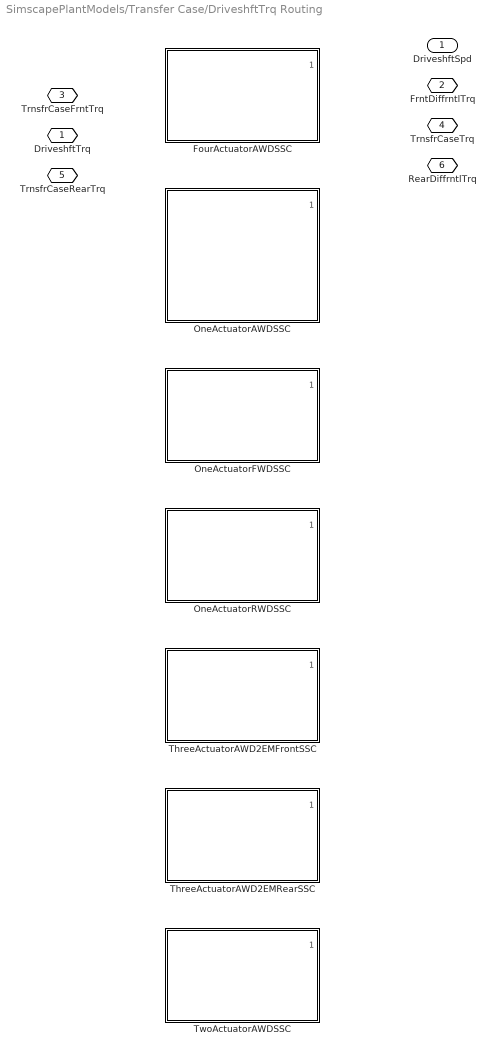
== system SimscapePlantModels/Transfer Case/DriveshftTrq Routing ==
  FourActuatorAWDSSC : Subsystem  VariantControl=FourActuatorAWDSSC  ReferencedSubsystem=FourActuatorAWDSSC
  OneActuatorAWDSSC : Subsystem  VariantControl=OneActuatorAWDSSC  ReferencedSubsystem=OneActuatorAWDSSC
  OneActuatorFWDSSC : Subsystem  VariantControl=OneActuatorFWDSSC  ReferencedSubsystem=OneActuatorFWDSSC
  OneActuatorRWDSSC : Subsystem  VariantControl=OneActuatorRWDSSC  ReferencedSubsystem=OneActuatorRWDSSC
  ThreeActuatorAWD2EMFrontSSC : Subsystem  VariantControl=ThreeActuatorAWD2EMFrontSSC  ReferencedSubsystem=ThreeActuatorAWD2EMFrontSSC
  ThreeActuatorAWD2EMRearSSC : Subsystem  VariantControl=ThreeActuatorAWD2EMRearSSC  ReferencedSubsystem=ThreeActuatorAWD2EMRearSSC
  TwoActuatorAWDSSC : Subsystem  VariantControl=TwoActuatorAWDSSC  ReferencedSubsystem=TwoActuatorAWDSSC
  DriveshftTrq : PMIOPort  Side=Left
  FrntDiffrntlTrq : PMIOPort  Port=2  Side=Right
  TrnsfrCaseFrntTrq : PMIOPort  Port=3  Side=Right
  TrnsfrCaseTrq : PMIOPort  Port=4  Side=Right
  TrnsfrCaseRearTrq : PMIOPort  Port=5  Side=Right
  RearDiffrntlTrq : PMIOPort  Port=6  Side=Right
  DriveshftSpd : Outport  VectorParamsAs1DForOutWhenUnconnected=off

== system SimscapePlantModels/Vehicle Body/IMu Sensor ==
  Veh : Inport
  IMUSensor : Subsystem  VariantControl=IMUSensor  ReferencedSubsystem=IMUSensor
  NoIMUSensor : Subsystem  VariantControl=NoIMUSensor  ReferencedSubsystem=NoIMUSensor
  IMU : Outport

== system SimscapePlantModels/Vehicle Body/Vehicle ==
  Env : Inport
  VehicleBody1DOFLongitudinalSSC : Subsystem  VariantControl=VehicleBody1DOFLongitudinalSSC  ReferencedSubsystem=VehicleBody1DOFLongitudinalSSC
  VehicleBody2DOFLongitudinalSSC : Subsystem  VariantControl=VehicleBody2DOFLongitudinalSSC  ReferencedSubsystem=VehicleBody2DOFLongitudinalSSC
  VehicleBody6DOFSSC : Subsystem  VariantControl=VehicleBody6DOFSSC  ReferencedSubsystem=VehicleBody6DOFSSC
  FrntAxlVeh : PMIOPort  Side=Left
  RearAxlVeh : PMIOPort  Port=2  Side=Left
  Solver : PMIOPort  Port=3  Side=Right
  VehBody : Outport

== system SimscapePlantModels/Pedals, Cluster, Cabin/Pedal, Cluster, Cabin/Brake Pedal ==
  DecelCmd : Inport
  Dead Zone1 : DeadZone  LowerValue=0  UpperValue=.01  ZeroCross=off
  DecelFdbk : Outport
  wires:
  Dead Zone1/1 -> DecelFdbk/1
  DecelCmd/1 -> Dead Zone1/1
